simulink model "Control_Con_Red_Neuronal"  (R2016a)
settings: Solver=VariableStepAuto  StartTime=0.0  StopTime=60  RelTol=1e-3
settings Model: Creator=Daniel  LastModifiedBy=Daniel

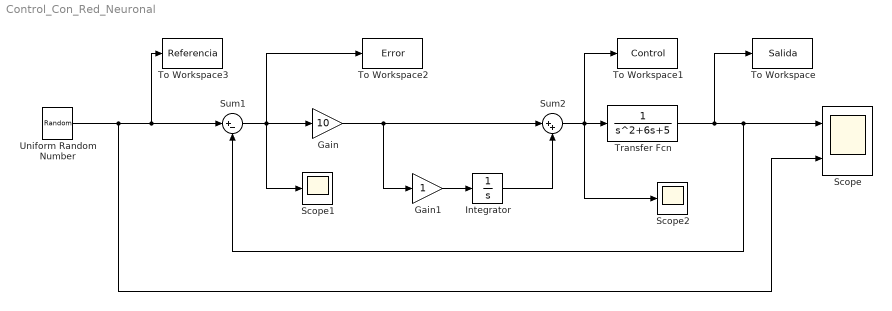
== system Control_Con_Red_Neuronal ==
  Gain : Gain  Gain=10
  Gain1 : Gain
  Integrator : Integrator
  Scope : Scope  NumInputPorts=2
  Scope1 : Scope
  Scope2 : Scope
  Sum1 : Sum  Inputs=|+-
  Sum2 : Sum  Inputs=|++
  To Workspace : ToWorkspace  VariableName=Salida  SampleTime=0.06
  To Workspace1 : ToWorkspace  VariableName=Control  SampleTime=0.06
  To Workspace2 : ToWorkspace  VariableName=Error  SampleTime=0.06
  To Workspace3 : ToWorkspace  VariableName=Referencia  SampleTime=0.06
  Transfer Fcn : TransferFcn  Denominator=[1 6 5]
  Uniform Random Number : UniformRandomNumber  Minimum=0  SampleTime=3
  wires:
  Sum1/1 -> Scope1/1, To Workspace2/1, Gain/1
  Gain/1 -> Gain1/1, Sum2/1
  Sum2/1 -> Scope2/1, Transfer Fcn/1, To Workspace1/1
  Integrator/1 -> Sum2/2
  Gain1/1 -> Integrator/1
  Transfer Fcn/1 -> To Workspace/1, Sum1/2, Scope/1
  Uniform Random Number/1 -> Scope/2, To Workspace3/1, Sum1/1
